simulink model "cap_estimation"  (R2015b)
settings: Solver=VariableStepAuto  StartTime=0.0  StopTime=10.0  RelTol=1e-3
libraries: elec_lib x18, fl_lib x16, nesl_utility x6
settings Model: Creator=Martin Andersen  LastModifiedBy=Martin Andersen

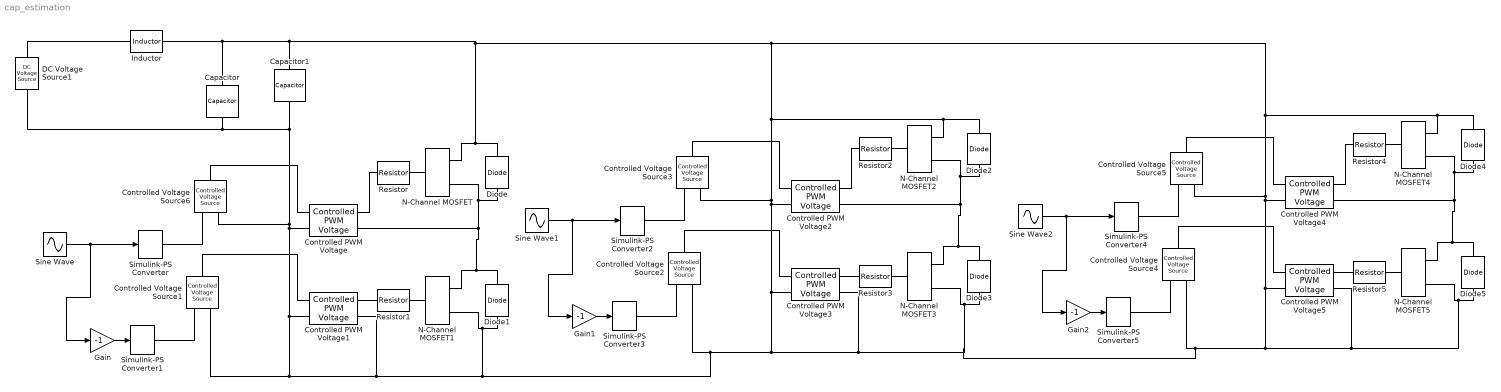
== system cap_estimation ==
  Capacitor : fl_lib/Electrical/Electrical Elements/Capacitor  c=8*2200e-6 F  r=.0125 Ohm  g=0 1/Ohm  i_specify=off  i_priority=None  i=0 A  v_specify=off  v_priority=None  v=0 V  vc_specify=off  vc_priority=None  vc=0 V
  Capacitor1 : fl_lib/Electrical/Electrical Elements/Capacitor  c=4.7e-6*8 F  r=1e-6 Ohm  g=0 1/Ohm  i_specify=off  i_priority=None  i=0 A  v_specify=off  v_priority=None  v=0 V  vc_specify=off  vc_priority=None  vc=0 V
  Controlled PWM Voltage{,1..5} (6 alike) : elec_lib/Actuators & Drivers/Drivers/Controlled PWM Voltage  F=20000 Hz  TD=0 s  pulse_width_offset=0 s  Vmin=-1 V  Vmax=1 V  Vm=10 V  pwm_or_av=1  event_type=1  sample_time=1e-6 s
  Controlled Voltage Source{1..6} (6 alike) : fl_lib/Electrical/Electrical Sources/Controlled Voltage Source
  DC Voltage Source1 : fl_lib/Electrical/Electrical Sources/DC Voltage Source  v0=52.8 V
  Diode{,1..5} (6 alike) : elec_lib/Semiconductor Devices/Diode  ModelType=3  Vf=0.6 V  Ron=0.3 Ohm  Goff=1e-8 S  Rz=0.3 Ohm  Vz=50 V  C_PWL=5 pF  prmExp=1  I12=[ 10 180*2 ] A  V12=[ 0.5 1.3 ] V  I1=0.0137 A  V1=0.6 V  RS=0.01 Ohm  IS=1e-12 A  Tmeas=25 C  ec=1  BV=Inf V  C_param=1  CJ0=5 pF  VJ=1 V  Mgrad=0.5  Vvec=[ 0.1 10 100 ] V  Cvec=[ 3.5 1 0.4 ] pF  FC=0.5  Q_param=1  Irrm=-7.15 A  iF=4 A  didt=-750 A/us  trr=115 ns  TT=50 ns  tau=100 ns  T_param=1  IS_T2=1.25e-7 A  I1_T2=0.245 A  V1_T2=0.5 V  Tmeas2=125 C  EG_param=1  EG=1.11 eV  XTI_param=1  XTI=3  dBVdT=0 V/K  Tdevice=25 C  Rth=[ 0 10 ] K/W  thermal_mass_parameterization=1  thermal_mass=[ 0 1 ] J/K  thermal_time_constant=[ 0 10 ] s  thermal_mass_initial_temperatures=[ 25 25 ] C
  Gain : Gain  Gain=-1
  Gain1 : Gain  Gain=-1
  Gain2 : Gain  Gain=-1
  Inductor : fl_lib/Electrical/Electrical Elements/Inductor  l=36e-6 H  r=1.9e-3 Ohm  g=1e-9 1/Ohm  i_specify=off  i_priority=None  i=0 A  v_specify=off  v_priority=None  v=0 V  i_L_specify=off  i_L_priority=None  i_L=0 A
  N-Channel MOSFET{,1..5} (6 alike) : elec_lib/Semiconductor Devices/N-Channel MOSFET  parameterization=1  prmDatasheet=1  prmEquCoeff=1  Beta=5 A/V^2  Rds=1e-3 Ohm  Id=390 A  Vgs=10 V  Vth=2 V  lam=0 1/V  Tmeas=25 C  RS=1e-4 Ohm  RD=0.01 Ohm  C_param=1  C_GS=270 pF  C_GD=80 pF  C_iss=19.86 nF  C_rss=540 pF  C_oss=1360 pF  C_GS_vec=[ 270 300 290 280 295 255 ] pF  C_GD_vec=[ 450 400 300 190 95 55 ] pF  C_iss_vec=[ 720 700 590 470 390 310 ] pF  C_rss_vec=[ 450 400 300 190 95 55 ] pF  C_oss_vec=[ 900 810 690 420 270 170 ] pF  C_Vds_vec=[ 0.1 0.3 1 3 10 30 ] V  charge_linearity_param=1  C_OX=200 pF  V_C_OX=-0.5 V  dVth_dT=-6 mV/K  Rds_T2=0.037 Ohm  Tmeas2=125 C  BEXDatasheet=-1.5  BEXEquCoeff=-1.5  TdeviceDatasheet=25 C  TdeviceEquCoeff=25 C  Rth=[ 0 10 ] K/W  thermal_mass_parameterization=1  thermal_mass=[ 0 1 ] J/K  thermal_time_constant=[ 0 10 ] s  thermal_mass_initial_temperatures=[ 25 25 ] C
  Resistor{,1..5} (6 alike) : fl_lib/Electrical/Electrical Elements/Resistor  R=4.5 Ohm  i_specify=off  i_priority=None  i=0 A  v_specify=off  v_priority=None  v=0 V
  Simulink-PS Converter{,1..5} (6 alike) : nesl_utility/Simulink-PS Converter  PhysicalDomain=network_engine_domain  SubClassName=ps_input  LeftPortType=input  RightPortType=output  PseudoPeriodic=off  Frequencies=[]  NoiseDistribution=none  NoiseParameters=[]  Unit=1  AffineConversion=off  InputFiltering=off  SimscapeFilterOrder=1  InputFilterTimeConstant=0.001  UdotUserProvided=1
  Sine Wave : Sin  Frequency=2*pi*5000  SampleTime=0
  Sine Wave1 : Sin  Frequency=2*pi*5000  SampleTime=0
  Sine Wave2 : Sin  Frequency=2*pi*5000  SampleTime=0
  wires:
  Sine Wave/1 -> Gain/1, Simulink-PS Converter/1
  Gain/1 -> Simulink-PS Converter1/1
  Sine Wave1/1 -> Simulink-PS Converter2/1, Gain1/1
  Gain1/1 -> Simulink-PS Converter3/1
  Sine Wave2/1 -> Gain2/1, Simulink-PS Converter4/1
  Gain2/1 -> Simulink-PS Converter5/1
  connections:
  Inductor/LConn1 -- DC Voltage Source1/LConn1
  Diode/LConn1 -- Controlled PWM Voltage/RConn2 -- N-Channel MOSFET1/RConn1 -- Diode1/RConn1 -- N-Channel MOSFET/RConn2
  Resistor/RConn1 -- N-Channel MOSFET/LConn1
  Resistor1/RConn1 -- N-Channel MOSFET1/LConn1
  Controlled PWM Voltage/RConn1 -- Resistor/LConn1
  Controlled Voltage Source6/LConn1 -- Controlled PWM Voltage/LConn1
  Simulink-PS Converter/RConn1 -- Controlled Voltage Source6/RConn1
  Controlled Voltage Source1/LConn1 -- Controlled PWM Voltage1/LConn1
  Simulink-PS Converter1/RConn1 -- Controlled Voltage Source1/RConn1
  Controlled PWM Voltage1/RConn1 -- Resistor1/LConn1
  Controlled PWM Voltage2/RConn2 -- Diode3/RConn1 -- N-Channel MOSFET3/RConn1 -- N-Channel MOSFET2/RConn2 -- Diode2/LConn1
  Controlled Voltage Source3/LConn1 -- Controlled PWM Voltage2/LConn1
  Simulink-PS Converter3/RConn1 -- Controlled Voltage Source2/RConn1
  Controlled Voltage Source2/LConn1 -- Controlled PWM Voltage3/LConn1
  Simulink-PS Converter2/RConn1 -- Controlled Voltage Source3/RConn1
  Controlled PWM Voltage2/RConn1 -- Resistor2/LConn1
  Controlled PWM Voltage3/RConn1 -- Resistor3/LConn1
  Resistor3/RConn1 -- N-Channel MOSFET3/LConn1
  Resistor2/RConn1 -- N-Channel MOSFET2/LConn1
  Diode5/RConn1 -- Diode4/LConn1 -- N-Channel MOSFET4/RConn2 -- Controlled PWM Voltage4/RConn2 -- N-Channel MOSFET5/RConn1
  Capacitor/RConn1 -- Capacitor1/RConn1 -- Controlled PWM Voltage1/LConn2 -- Controlled PWM Voltage1/RConn2 -- Controlled PWM Voltage3/LConn2 -- Controlled PWM Voltage2/LConn2 -- N-Channel MOSFET/RConn1 -- Diode/RConn1 -- Inductor/RConn1 -- Capacitor/LConn1 -- Capacitor1/LConn1 -- Diode4/RConn1 -- N-Channel MOSFET4/RConn1 -- Controlled Voltage Source4/RConn2 -- Diode5/LConn1 -- N-Channel MOSFET5/RConn2 -- Controlled PWM Voltage5/RConn2 -- Controlled PWM Voltage5/LConn2 -- Controlled PWM Voltage4/LConn2 -- Controlled Voltage Source5/RConn2 -- Diode2/RConn1 -- N-Channel MOSFET2/RConn1 -- Controlled Voltage Source3/RConn2 -- Controlled PWM Voltage3/RConn2 -- N-Channel MOSFET3/RConn2 -- Diode3/LConn1 -- Controlled Voltage Source2/RConn2 -- Diode1/LConn1 -- N-Channel MOSFET1/RConn2 -- Controlled Voltage Source1/RConn2 -- Controlled PWM Voltage/LConn2 -- Controlled Voltage Source6/RConn2 -- DC Voltage Source1/RConn1
  Controlled Voltage Source5/LConn1 -- Controlled PWM Voltage4/LConn1
  Controlled PWM Voltage5/RConn1 -- Resistor5/LConn1
  Controlled Voltage Source4/LConn1 -- Controlled PWM Voltage5/LConn1
  Resistor4/RConn1 -- N-Channel MOSFET4/LConn1
  Simulink-PS Converter5/RConn1 -- Controlled Voltage Source4/RConn1
  Resistor5/RConn1 -- N-Channel MOSFET5/LConn1
  Controlled PWM Voltage4/RConn1 -- Resistor4/LConn1
  Simulink-PS Converter4/RConn1 -- Controlled Voltage Source5/RConn1
